simulink model "t_4"  (R2023b)
settings: Solver=VariableStepAuto  StartTime=0.0  StopTime=10.0  RelTol=1e-3
settings Model: Creator=86186  LastModifiedBy=86186

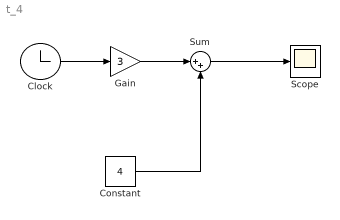
== system t_4 ==
  Clock : Clock
  Constant : Constant  Value=4
  Gain : Gain  Gain=3
  Scope : Scope
  Sum : Sum  Inputs=|++
  wires:
  Clock/1 -> Gain/1
  Gain/1 -> Sum/1
  Constant/1 -> Sum/2
  Sum/1 -> Scope/1
